simulink model "XY_Gantry_Simulink"  (R2022a)
settings: Solver=ode14x  StartTime=0.0  StopTime=0.01  FixedStep=1e-3  MaxStep=1e-3  RelTol=1e-3
values from neighbouring files (symbols this model uses):
  B = 0.1    [XY_Gantry_Matlab.m]    (also in XY_Gantry_Matlab2.m = 0.001)
  D = 4*2.4525    (= 9.81)    [XY_Gantry_Matlab.m]    (also in XY_Gantry_Matlab2.m)
  g = 9.81    [XY_Gantry_Matlab.m]    (also in XY_Gantry_Matlab2.m)
  J = 0.1e-4    (= 1e-05)    [XY_Gantry_Matlab.m]    (also in XY_Gantry_Matlab2.m)
  K = 4*6.5    (= 26)    [XY_Gantry_Matlab.m]    (also in XY_Gantry_Matlab2.m)
  Ls = 3.7e-3    (= 0.0037)    [XY_Gantry_Matlab.m]    (also in XY_Gantry_Matlab2.m)
  m = 2    [XY_Gantry_Matlab.m]    (also in XY_Gantry_Matlab2.m)
  M = 0.5    [XY_Gantry_Matlab.m]    (also in XY_Gantry_Matlab2.m)
  p = 360/(2*m*step)    [XY_Gantry_Matlab.m]    (also in XY_Gantry_Matlab2.m = 50)
  r = 6e-3    (= 0.006)    [XY_Gantry_Matlab.m]    (also in XY_Gantry_Matlab2.m)
  Rs = 1.1    [XY_Gantry_Matlab.m]    (also in XY_Gantry_Matlab2.m)
settings Model: Creator=lenovo  LastModifiedBy=lenovo

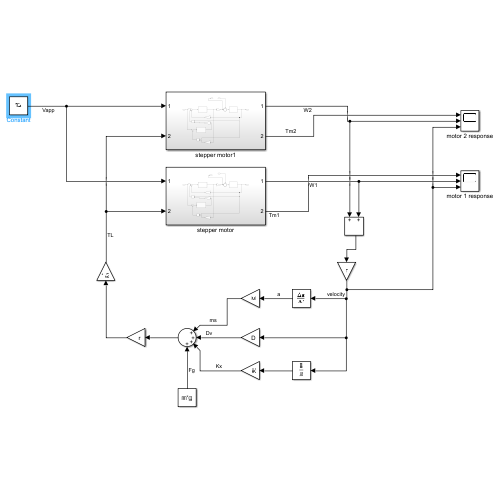
[thumbnail: Simulink's stored preview of the top-level diagram]
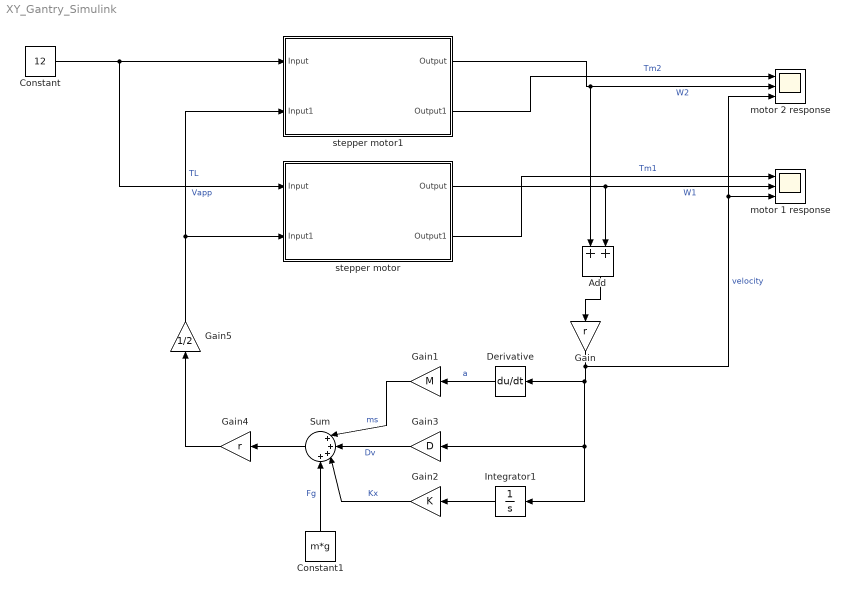
== system XY_Gantry_Simulink ==
  Add : Sum
  Constant : Constant  Value=12
  Constant1 : Constant  Value=m*g
  Derivative : Derivative
  Gain : Gain  Gain=r
  Gain1 : Gain  Gain=M
  Gain2 : Gain  Gain=K
  Gain3 : Gain  Gain=D
  Gain4 : Gain  Gain=r
  Gain5 : Gain  Gain=1/2
  Integrator1 : Integrator
  Sum : Sum  Inputs=|++++
  motor 1 response : Scope  NumInputPorts=3
  motor 2 response : Scope  NumInputPorts=3
  stepper motor : Subsystem
  stepper motor1 : Subsystem
  wires:
  stepper motor/1(Output) -> Add/2, motor 1 response/2  "W1"
  Gain/1 -> motor 2 response/3, motor 1 response/3, Gain3/1, Integrator1/1, Derivative/1  "velocity"
  Derivative/1 -> Gain1/1  "a"
  Integrator1/1 -> Gain2/1
  Gain1/1 -> Sum/1  "ms"
  Gain3/1 -> Sum/2  "Dv"
  Gain2/1 -> Sum/3  "Kx"
  Constant1/1 -> Sum/4  "Fg"
  Sum/1 -> Gain4/1
  Gain4/1 -> Gain5/1
  Gain5/1 -> stepper motor1/2(Input1), stepper motor/2(Input1)  "TL"
  Add/1 -> Gain/1
  stepper motor1/1(Output) -> motor 2 response/2, Add/1  "W2"
  Constant/1 -> stepper motor/1(Input), stepper motor1/1(Input)  "Vapp"
  stepper motor1/2(Output1) -> motor 2 response/1  "Tm2"
  stepper motor/2(Output1) -> motor 1 response/1  "Tm1"

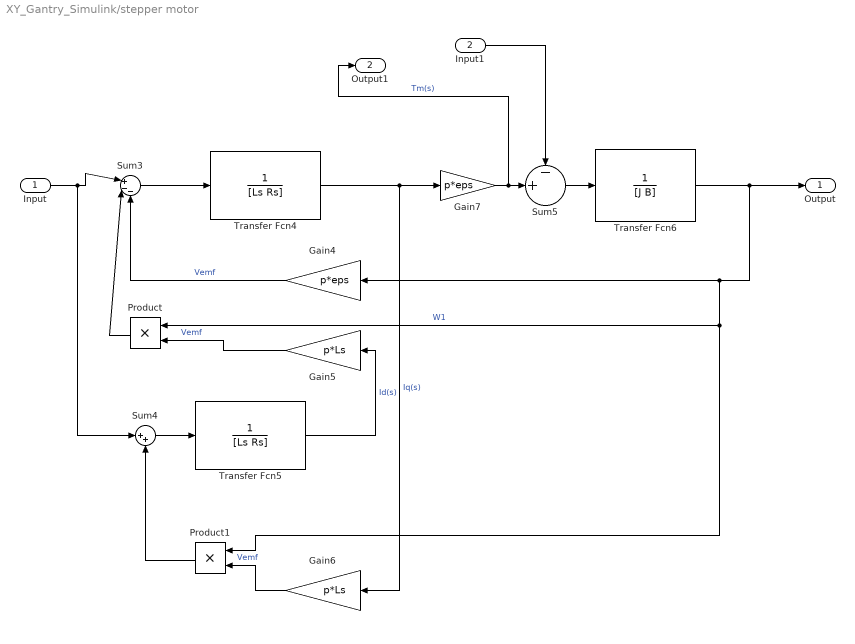
== system XY_Gantry_Simulink/stepper motor ==
  Input : Inport
  Input1 : Inport  Port=2
  Gain4 : Gain  Gain=p*eps
  Gain5 : Gain  Gain=p*Ls
  Gain6 : Gain  Gain=p*Ls
  Gain7 : Gain  Gain=p*eps
  Product : Product
  Product1 : Product
  Sum3 : Sum  Inputs=|+--
  Sum4 : Sum  Inputs=|++
  Sum5 : Sum  Inputs=-+|
  Transfer Fcn4 : TransferFcn  Denominator=[Ls Rs]
  Transfer Fcn5 : TransferFcn  Denominator=[Ls Rs]
  Transfer Fcn6 : TransferFcn  Denominator=[J B]
  Output : Outport
  Output1 : Outport  Port=2
  wires:
  Transfer Fcn5/1 -> Gain5/1  "Id(s)"
  Transfer Fcn4/1 -> Gain7/1, Gain6/1  "Iq(s)"
  Sum4/1 -> Transfer Fcn5/1
  Gain4/1 -> Sum3/3  "Vemf"
  Sum3/1 -> Transfer Fcn4/1
  Transfer Fcn6/1 -> Output/1, Product/1, Product1/1, Gain4/1  "W1"
  Gain5/1 -> Product/2  "Vemf"
  Product/1 -> Sum3/2
  Gain6/1 -> Product1/2  "Vemf"
  Product1/1 -> Sum4/2
  Input/1 -> Sum4/1, Sum3/1
  Input1/1 -> Sum5/1
  Gain7/1 -> Output1/1, Sum5/2  "Tm(s)"
  Sum5/1 -> Transfer Fcn6/1

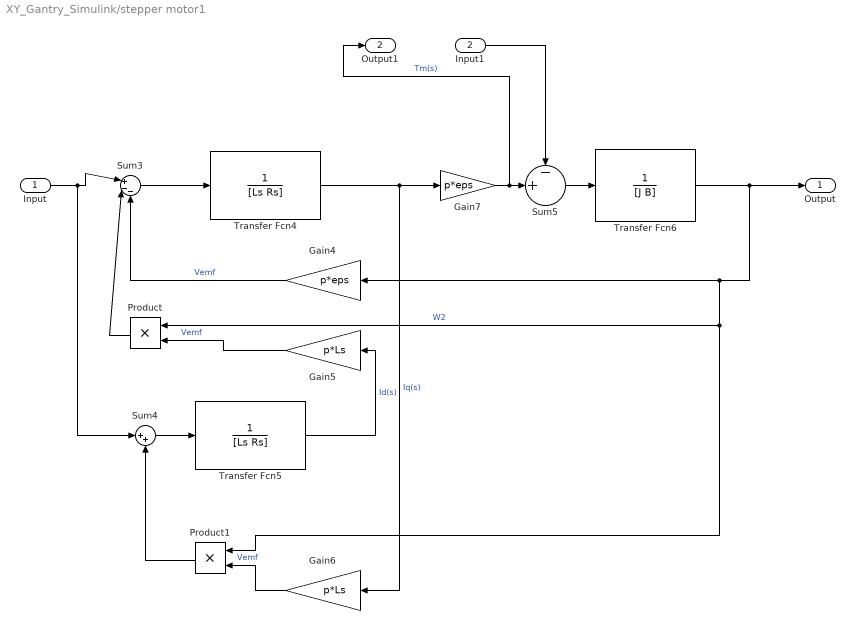
== system XY_Gantry_Simulink/stepper motor1 ==
  Input : Inport
  Input1 : Inport  Port=2
  Gain4 : Gain  Gain=p*eps
  Gain5 : Gain  Gain=p*Ls
  Gain6 : Gain  Gain=p*Ls
  Gain7 : Gain  Gain=p*eps
  Product : Product
  Product1 : Product
  Sum3 : Sum  Inputs=|+--
  Sum4 : Sum  Inputs=|++
  Sum5 : Sum  Inputs=-+|
  Transfer Fcn4 : TransferFcn  Denominator=[Ls Rs]
  Transfer Fcn5 : TransferFcn  Denominator=[Ls Rs]
  Transfer Fcn6 : TransferFcn  Denominator=[J B]
  Output : Outport
  Output1 : Outport  Port=2
  wires:
  Transfer Fcn5/1 -> Gain5/1  "Id(s)"
  Transfer Fcn4/1 -> Gain7/1, Gain6/1  "Iq(s)"
  Sum4/1 -> Transfer Fcn5/1
  Gain4/1 -> Sum3/3  "Vemf"
  Sum3/1 -> Transfer Fcn4/1
  Transfer Fcn6/1 -> Output/1, Product/1, Product1/1, Gain4/1  "W2"
  Gain5/1 -> Product/2  "Vemf"
  Product/1 -> Sum3/2
  Gain6/1 -> Product1/2  "Vemf"
  Product1/1 -> Sum4/2
  Input/1 -> Sum4/1, Sum3/1
  Input1/1 -> Sum5/1
  Gain7/1 -> Output1/1, Sum5/2  "Tm(s)"
  Sum5/1 -> Transfer Fcn6/1
